simulink model "double_pend_simulation"  (R2021a)
settings: Solver=VariableStepAuto  StartTime=0.0  StopTime=stoptime  RelTol=1e-7
values from neighbouring files (symbols this model uses):
  frequency = 2    [rundoublesim.m]
  I1 = 0.1*(0.1^2+0.0254^2)/12+0.2*l1^2/2+0.2*R1^2    (= 0.0504180596667)    [rundoublesim.m]
  I2 = 0.1*(0.1^2+0.0254^2)/12    (= 8.87096666667e-05)    [rundoublesim.m]
  l1 = 0.459    [rundoublesim.m]
  m1 = 0.3    [rundoublesim.m]
  m2 = 0.1    [rundoublesim.m]
  mc = 0.3    [rundoublesim.m]
  R1 = (0.1*l1/2+l1*0.2)/0.3    (= 0.3825)    [rundoublesim.m]
  R2 = 0.459/2    (= 0.2295)    [rundoublesim.m]
  theta1_0 = idx    [rundoublesim.m]
  theta2_0 = jdx    [rundoublesim.m]
settings Model: Creator=natha  LastModifiedBy=natha
settings DebuggingCC: AlgebraicLoopMsg=none

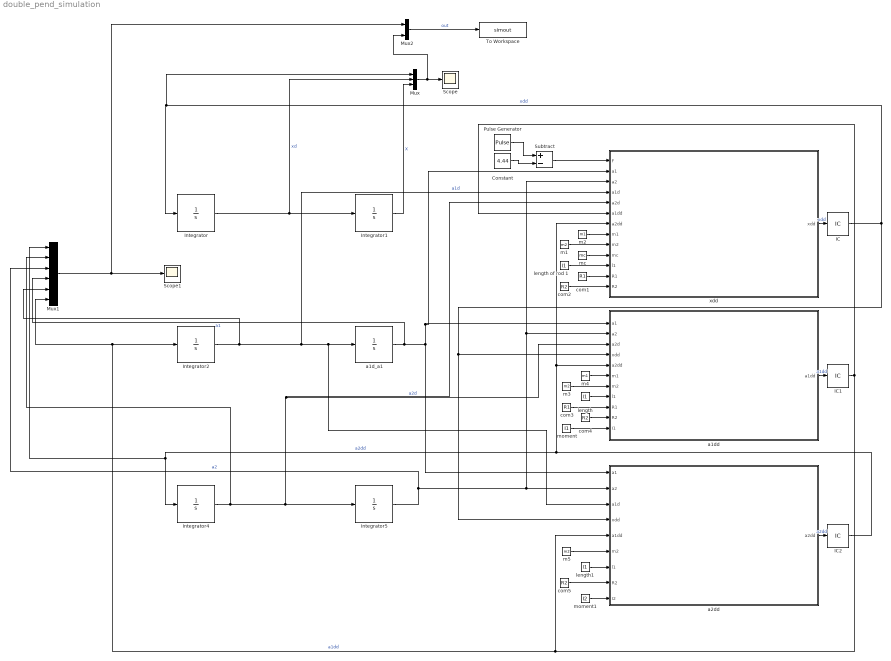
== system double_pend_simulation ==
  Constant : Constant  Value=4.44
  IC : InitialCondition  Value=0
  IC1 : InitialCondition  Value=0
  IC2 : InitialCondition  Value=0
  Integrator{,1..2,4} (4 alike) : Integrator
  Integrator5 : Integrator  InitialCondition=theta2_0
  Mux : Mux  Inputs=3
  Mux1 : Mux  Inputs=6
  Mux2 : Mux  Inputs=2
  Pulse Generator : DiscretePulseGenerator  PulseType=Time based  Amplitude=8.88  Period=1/frequency  PulseWidth=50
  Scope : Scope
  Scope1 : Scope
  Subtract : Sum  Inputs=+-
  To Workspace : ToWorkspace  VariableName=simout  SaveFormat=Timeseries  SampleTime=-1
  a1d_a1 : Integrator  InitialCondition=theta1_0
  a1dd : MATLAB Function  TreatAsAtomicUnit=on
  a2dd : MATLAB Function  TreatAsAtomicUnit=on
  com1 : Constant  Value=R1
  com2 : Constant  Value=R2
  com3 : Constant  Value=R1
  com4 : Constant  Value=R2
  com5 : Constant  Value=R2
  length : Constant  Value=l1
  length of rod 1 : Constant  Value=l1
  length1 : Constant  Value=l1
  m1 : Constant  Value=m2
  m2 : Constant  Value=m1
  m3 : Constant  Value=m2
  m4 : Constant  Value=m1
  m5 : Constant  Value=m2
  mc : Constant  Value=mc
  moment : Constant  Value=I1
  moment1 : Constant  Value=I2
  xdd : MATLAB Function  TreatAsAtomicUnit=on
  wires:
  length of rod 1/1 -> xdd/11(l1)
  com1/1 -> xdd/12(R1)
  com2/1 -> xdd/13(R2)
  mc/1 -> xdd/10(mc)
  m1/1 -> xdd/9(m2)
  m2/1 -> xdd/8(m1)
  Subtract/1 -> xdd/1(F)
  com4/1 -> a1dd/10(R2)
  com3/1 -> a1dd/9(R1)
  length/1 -> a1dd/8(l1)
  m3/1 -> a1dd/7(m2)
  m4/1 -> a1dd/6(m1)
  moment/1 -> a1dd/11(I1)
  m5/1 -> a2dd/6(m2)
  length1/1 -> a2dd/7(l1)
  com5/1 -> a2dd/8(R2)
  moment1/1 -> a2dd/9(I2)
  IC2/1 -> a1dd/5(a2dd), xdd/7(a2dd), Mux1/1, Integrator4/1  "a2dd"
  Integrator4/1 -> Mux1/2, xdd/5(a2d), a1dd/3(a2d), Integrator5/1  "a2d"
  Integrator5/1 -> Mux1/3, xdd/3(a2), a1dd/2(a2), a2dd/2(a2)  "a2"
  IC/1 -> a1dd/4(xdd), a2dd/4(xdd), Mux/1, Integrator/1  "xdd"
  IC1/1 -> Mux1/6, Integrator2/1, a2dd/5(a1dd), xdd/6(a1dd)  "a1dd"
  Integrator2/1 -> Mux1/5, xdd/4(a1d), a2dd/3(a1d), a1d_a1/1  "a1d"
  a1d_a1/1 -> Mux1/4, a2dd/1(a1), xdd/2(a1), a1dd/1(a1)  "a1"
  Integrator/1 -> Mux/2, Integrator1/1  "xd"
  Integrator1/1 -> Mux/3  "X"
  Mux/1 -> Mux2/2, Scope/1
  Mux1/1 -> Mux2/1, Scope1/1
  xdd/1(xdd) -> IC/1  "xdd"
  a1dd/1(a1dd) -> IC1/1  "a1dd"
  a2dd/1(a2dd) -> IC2/1  "a2dd"
  Mux2/1 -> To Workspace/1  "out"
  Pulse Generator/1 -> Subtract/1
  Constant/1 -> Subtract/2

== matlab function double_pend_simulation/a1dd ==
  data: a1 input; a1dd output; a2 input; a2d input; xdd input; a2dd input; m1 input; m2 input; l1 input; R1 input; R2 input; I1 input
function a1dd  = a1doubledot(a1,a2,a2d,xdd,a2dd,m1,m2,l1,R1,R2,I1)
%calculates the angle 1 double dot term givin the other variables
    s1 = sin(a1);
    s2 = sin(a2);
    c1 = cos(a1);
    c2 = cos(a2);
    sig2=a2d^2;
    sig3=s1^2;
    sig4=c1^2;
    sig5 = xdd;
    sig6 = a2dd;
    g=9.806;
    denom = -(I1+R1^2*m1*sig4+R1^2*m1*sig3+l1^2*m2*sig4+l1^2*m2*sig3);
    num = R1*m1*c1*sig5+ l1*m2*c1*sig5 + R1*g*m1*s1 + g*l1*m2*s1 - R2*l1*m2*c1*s2*sig2 + R2*l1*m2*c2*s1*sig2 + R2*l1*m2*c1*c2*sig6 + R2*l1*m2*s1*s2*sig6;
    a1dd=num/denom;
end

== matlab function double_pend_simulation/xdd ==
  data: F input; xdd output; a1 input; a2 input; a1d input; a2d input; a1dd input; a2dd input; m1 input; m2 input; mc input; l1 input; R1 input; R2 input
function xdd  = xdoubledot(F,a1,a2,a1d,a2d,a1dd,a2dd,m1,m2,mc,l1,R1,R2)
%calculates the x double dot term givin the other variables
m=m1+m2+mc;
sig2 = a1d^2;
s1 = sin(a1);
s2 = sin(a2);
c1 = cos(a1);
c2 = cos(a2);

num=(-F)-R1*m1*s1*sig2-R2*m2*s2*a2d^2+R1*m1*c1*a1dd+R2*m2*c2*a2dd-l1*m2*s1*sig2+l1*m2*c1*a1dd;
xdd=-num/m;

end

== matlab function double_pend_simulation/a2dd ==
  data: a1 input; a2dd output; a2 input; a1d input; xdd input; a1dd input; m2 input; l1 input; R2 input; I2 input
function a2dd  = a2doubledot(a1,a2,a1d,xdd,a1dd,m2,l1,R2,I2)
%calculates the angle 2 double dot term givin the other variables
    s1 = sin(a1);
    s2 = sin(a2);
    c1 = cos(a1);
    c2 = cos(a2);
    sig2=a1d^2;
    sig3=a1dd;
    g=9.806;
    denom =-(I2+R2^2*m2*c2^2+R2^2*m2*s2^2);
    num = R2*m2*c2*xdd+R2*g*m2*s2+R2*l1*m2*c1*s2*sig2-R2*l1*m2*c2*s1*sig2+R2*l1*m2*c1*c2*sig3+R2*l1*m2*s1*s2*sig3;
    a2dd=num/denom;
end
